simulink model "sflib"  (Simulink 6.0)
settings: Solver=ode45  SolverMode=SingleTasking  StartTime=0.0  StopTime=10.0  RelTol=1e-3  AbsTol=1e-6
settings Model: Creator=The MathWorks Inc.  LastModifiedBy=batserve  ExtModeTrigMode=oneshot  ExtModeArmWhenConnect=off  ExtModeAutoUpdateStatusClock=off
settings DataIOCC: LimitDataPoints=off  SignalLoggingName=logsOut
settings OptimizationCC: BooleanDataType=off
settings DebuggingCC: CheckExecutionContextPreStartOutputMsg=on  CheckExecutionContextRuntimeOutputMsg=on  SolverPrmCheckMsg=none  IntegerOverflowMsg=none
settings HardwareCC: TargetUnknown=on
settings ModelReferenceCC: UpdateModelReferenceTargets=IfOutOfDate

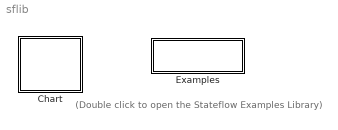
== system sflib ==
  note: (Double click to open the
      | Stateflow Examples Library)
  Chart : Stateflow chart  PropExecContextAcrossSSBoundary=on
  Examples : Subsystem  PropExecContextAcrossSSBoundary=on
      settings: OpenFcn=sf('Private','sf_examples')
      mask Display: disp('Examples')

== system sflib/Examples ==

== stateflow chart Chart ==
